simulink model "simulacion"  (R2019a)
settings: Solver=VariableStepAuto  StartTime=0.0  StopTime=25  RelTol=1e-3
values from neighbouring files (symbols this model uses):
  A = [1 -1.57039885123 1.27561332498 -0.484403368335 0.0761970646103]    [filtro.mat]
  B = [0.0185630106269 0.0742520425076 0.111378063761 0.0742520425076 0.0185630106269]    [filtro.mat]
  tm = 1.25531256352    [data_lineal.mat]    (also in modelo_1_orden_tiempo_muerto.m = 1.2620*dt25 - 0.2620*dt75; planta.mat)
libraries: cstblocks x17, simulink x9
settings Model: Creator=Juan P Velandia  LastModifiedBy=Juan P Velandia

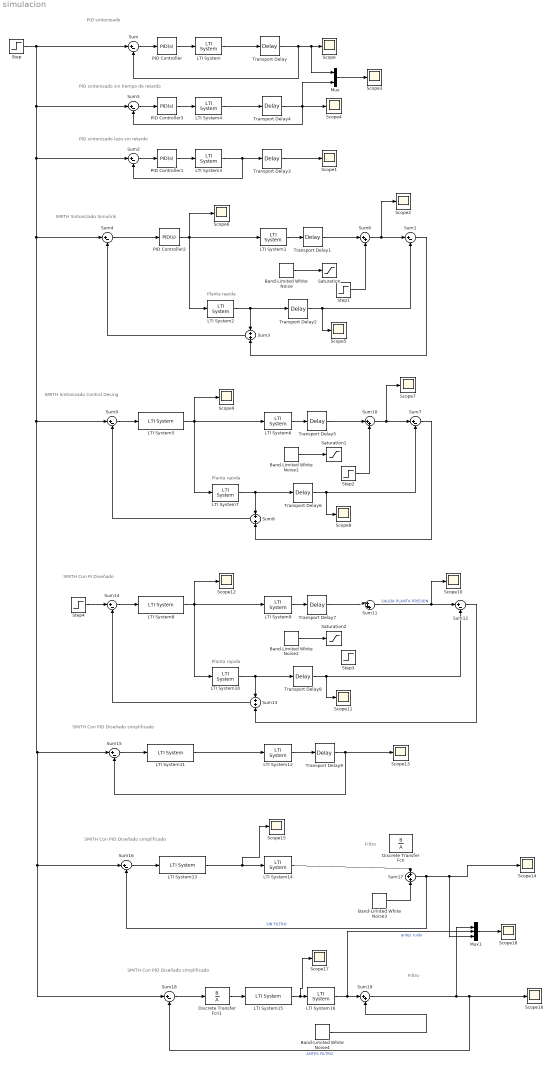
== system simulacion ==
  note: Filtro
  note: Planta rapida
  note: PID sintonizado
  note: PID sintonizado lazo sin retardo
  note: SMITH Sintonizado Simulink
  note: PID sintonizado sin tiempo de retardo
  note: Planta rapida
  note: SMITH Sintonizado Control Desing
  note: SMITH Con PI Diseñado
  note: Planta rapida
  note: SMITH Con PID Diseñado simplificado
  note: SMITH Con PID Diseñado simplificado
  note: Filtro
  note: SMITH Con PID Diseñado simplificado
  Band-Limited White Noise : simulink/Sources/Band-Limited White Noise  Cov=[0.1]  Ts=1  seed=[23341]
  Band-Limited White Noise1 : simulink/Sources/Band-Limited White Noise  Cov=[0.1]  Ts=1  seed=[23341]
  Band-Limited White Noise2 : simulink/Sources/Band-Limited White Noise  Cov=[0.1]  Ts=1  seed=[23341]
  Band-Limited White Noise3 : simulink/Sources/Band-Limited White Noise  Cov=[0.0008]  Ts=0.4  seed=[23341]
  Band-Limited White Noise4 : simulink/Sources/Band-Limited White Noise  Cov=[0.0008]  Ts=0.4  seed=[23341]
  Discrete Transfer Fcn : DiscreteTransferFcn  Numerator=B  Denominator=A
  Discrete Transfer Fcn1 : DiscreteTransferFcn  Numerator=B  Denominator=A
  LTI System{,1..2,6..7,9..10,12} (8 alike) : cstblocks/LTI System  sys=G  IC=[]
  LTI System11 : cstblocks/LTI System  sys=ceq  IC=[]
  LTI System13 : cstblocks/LTI System  sys=ceq_d  IC=[]
  LTI System14 : cstblocks/LTI System  sys=G_d  IC=[]
  LTI System15 : cstblocks/LTI System  sys=ceq_d  IC=[]
  LTI System16 : cstblocks/LTI System  sys=G_d  IC=[]
  LTI System3 : cstblocks/LTI System  sys=Gp1  IC=[]
  LTI System4 : cstblocks/LTI System  sys=Gp1  IC=[]
  LTI System5 : cstblocks/LTI System  sys=C  IC=[]
  LTI System8 : cstblocks/LTI System  sys=PI  IC=[]
  Mux : Mux  Inputs=2
  Mux1 : Mux  Inputs=3
  PID Controller : simulink/Continuous/PID Controller  Controller=PID  Form=Parallel  TimeDomain=Continuous-time  SampleTime=-1  IntegratorMethod=Forward Euler  FilterMethod=Forward Euler  ControllerParametersSource=internal  P=4249.87443519566  I=716.116002525779  D=-20348.5974264342  UseFilter=on  N=0.10676453447151  TunerSelectOption=Transfer Function Based (PID Tuner App)  InitialConditionSource=internal  InitialConditionForIntegrator=0  InitialConditionForFilter=0  DifferentiatorICPrevScaledInput=0  ExternalReset=none  TrackingMode=off  Kt=1  LimitOutput=off  UpperSaturationLimit=inf  LowerSaturationLimit=-inf  LinearizeAsGain=on  AntiWindupMode=none  Kb=1  POutMin=[]  POutMax=[]  IOutMin=[]  IOutMax=[]  DOutMin=[]  DOutMax=[]  NOutMin=[]  NOutMax=[]  SumOutMin=[]  SumOutMax=[]  SaturationOutMin=[]  SaturationOutMax=[]  PParamMin=[]  PParamMax=[]  IParamMin=[]  IParamMax=[]  DParamMin=[]  DParamMax=[]  NParamMin=[]  NParamMax=[]  KbParamMin=[]  KbParamMax=[]  KtParamMin=[]  KtParamMax=[]  KbOutMin=[]  KbOutMax=[]  KtOutMin=[]  KtOutMax=[]  IntegratorOutMin=[]  IntegratorOutMax=[]  FilterOutMin=[]  FilterOutMax=[]  SumI1OutMin=[]  SumI1OutMax=[]  SumI2OutMin=[]  SumI2OutMax=[]  SumI3OutMin=[]  SumI3OutMax=[]  SumI4OutMin=[]  SumI4OutMax=[]  SumDOutMin=[]  SumDOutMax=[]  DifferentiatorOutMin=[]  DifferentiatorOutMax=[]  FilterDiffOutCoefMin=[]  FilterDiffOutCoefMax=[]  ReciprocalOutMin=[]  ReciprocalOutMax=[]  SumDenOutMin=[]  SumDenOutMax=[]  SumNumOutMin=[]  SumNumOutMax=[]  DivideOutMin=[]  DivideOutMax=[]  IntegratorContinuousStateAttributes=''  IntegratorStateMustResolveToSignalObject=off  IntegratorRTWStateStorageClass=Auto  FilterContinuousStateAttributes=''  FilterStateMustResolveToSignalObject=off  FilterRTWStateStorageClass=Auto  ParallelPVariant=InternalParameters  IdealPVariant=Disabled  IVariant=InternalParameters  DVariant=InternalParameters  IntegratorVariant=Continuous  SatVariant=Disabled  AWVariant=Passthrough  PCopyVariant=Disabled  TRVariant=Disabled  FdbkBlocksVariant=Forward  IdealPFdbkVariant=Disabled  SatFdbkVariant=Disabled  DerivativeFilterVariant=ContFilter  NVariant=InternalParameters  NCopyVariant=Disabled  FilterICVariant=InternalICsFilter  IntegratorICVariant=InternalICs  ExternalResetVariant=Disabled  TRSumVariant=Passthrough  SumFdbkVariant=Disabled  SumVariant=Sum_PID
  PID Controller1 : simulink/Continuous/PID Controller  Controller=PID  Form=Parallel  TimeDomain=Continuous-time  SampleTime=-1  IntegratorMethod=Forward Euler  FilterMethod=Forward Euler  ControllerParametersSource=internal  P=5039.29122623723  I=1577.25793330017  D=-3349.52827806109  UseFilter=on  N=0.2130232522062  TunerSelectOption=Transfer Function Based (PID Tuner App)  InitialConditionSource=internal  InitialConditionForIntegrator=0  InitialConditionForFilter=0  DifferentiatorICPrevScaledInput=0  ExternalReset=none  TrackingMode=off  Kt=1  LimitOutput=off  UpperSaturationLimit=inf  LowerSaturationLimit=-inf  LinearizeAsGain=on  AntiWindupMode=none  Kb=1  POutMin=[]  POutMax=[]  IOutMin=[]  IOutMax=[]  DOutMin=[]  DOutMax=[]  NOutMin=[]  NOutMax=[]  SumOutMin=[]  SumOutMax=[]  SaturationOutMin=[]  SaturationOutMax=[]  PParamMin=[]  PParamMax=[]  IParamMin=[]  IParamMax=[]  DParamMin=[]  DParamMax=[]  NParamMin=[]  NParamMax=[]  KbParamMin=[]  KbParamMax=[]  KtParamMin=[]  KtParamMax=[]  KbOutMin=[]  KbOutMax=[]  KtOutMin=[]  KtOutMax=[]  IntegratorOutMin=[]  IntegratorOutMax=[]  FilterOutMin=[]  FilterOutMax=[]  SumI1OutMin=[]  SumI1OutMax=[]  SumI2OutMin=[]  SumI2OutMax=[]  SumI3OutMin=[]  SumI3OutMax=[]  SumI4OutMin=[]  SumI4OutMax=[]  SumDOutMin=[]  SumDOutMax=[]  DifferentiatorOutMin=[]  DifferentiatorOutMax=[]  FilterDiffOutCoefMin=[]  FilterDiffOutCoefMax=[]  ReciprocalOutMin=[]  ReciprocalOutMax=[]  SumDenOutMin=[]  SumDenOutMax=[]  SumNumOutMin=[]  SumNumOutMax=[]  DivideOutMin=[]  DivideOutMax=[]  IntegratorContinuousStateAttributes=''  IntegratorStateMustResolveToSignalObject=off  IntegratorRTWStateStorageClass=Auto  FilterContinuousStateAttributes=''  FilterStateMustResolveToSignalObject=off  FilterRTWStateStorageClass=Auto  ParallelPVariant=InternalParameters  IdealPVariant=Disabled  IVariant=InternalParameters  DVariant=InternalParameters  IntegratorVariant=Continuous  SatVariant=Disabled  AWVariant=Passthrough  PCopyVariant=Disabled  TRVariant=Disabled  FdbkBlocksVariant=Forward  IdealPFdbkVariant=Disabled  SatFdbkVariant=Disabled  DerivativeFilterVariant=ContFilter  NVariant=InternalParameters  NCopyVariant=Disabled  FilterICVariant=InternalICsFilter  IntegratorICVariant=InternalICs  ExternalResetVariant=Disabled  TRSumVariant=Passthrough  SumFdbkVariant=Disabled  SumVariant=Sum_PID
  PID Controller2 : simulink/Continuous/PID Controller  Controller=PID  Form=Parallel  TimeDomain=Continuous-time  SampleTime=-1  IntegratorMethod=Forward Euler  FilterMethod=Forward Euler  ControllerParametersSource=internal  P=5039.29122623723  I=1577.25793330017  D=-3349.52827806109  UseFilter=on  N=0.2130232522062  TunerSelectOption=Transfer Function Based (PID Tuner App)  InitialConditionSource=internal  InitialConditionForIntegrator=0  InitialConditionForFilter=0  DifferentiatorICPrevScaledInput=0  ExternalReset=none  TrackingMode=off  Kt=1  LimitOutput=off  UpperSaturationLimit=inf  LowerSaturationLimit=-inf  LinearizeAsGain=on  AntiWindupMode=none  Kb=1  POutMin=[]  POutMax=[]  IOutMin=[]  IOutMax=[]  DOutMin=[]  DOutMax=[]  NOutMin=[]  NOutMax=[]  SumOutMin=[]  SumOutMax=[]  SaturationOutMin=[]  SaturationOutMax=[]  PParamMin=[]  PParamMax=[]  IParamMin=[]  IParamMax=[]  DParamMin=[]  DParamMax=[]  NParamMin=[]  NParamMax=[]  KbParamMin=[]  KbParamMax=[]  KtParamMin=[]  KtParamMax=[]  KbOutMin=[]  KbOutMax=[]  KtOutMin=[]  KtOutMax=[]  IntegratorOutMin=[]  IntegratorOutMax=[]  FilterOutMin=[]  FilterOutMax=[]  SumI1OutMin=[]  SumI1OutMax=[]  SumI2OutMin=[]  SumI2OutMax=[]  SumI3OutMin=[]  SumI3OutMax=[]  SumI4OutMin=[]  SumI4OutMax=[]  SumDOutMin=[]  SumDOutMax=[]  DifferentiatorOutMin=[]  DifferentiatorOutMax=[]  FilterDiffOutCoefMin=[]  FilterDiffOutCoefMax=[]  ReciprocalOutMin=[]  ReciprocalOutMax=[]  SumDenOutMin=[]  SumDenOutMax=[]  SumNumOutMin=[]  SumNumOutMax=[]  DivideOutMin=[]  DivideOutMax=[]  IntegratorContinuousStateAttributes=''  IntegratorStateMustResolveToSignalObject=off  IntegratorRTWStateStorageClass=Auto  FilterContinuousStateAttributes=''  FilterStateMustResolveToSignalObject=off  FilterRTWStateStorageClass=Auto  ParallelPVariant=InternalParameters  IdealPVariant=Disabled  IVariant=InternalParameters  DVariant=InternalParameters  IntegratorVariant=Continuous  SatVariant=Disabled  AWVariant=Passthrough  PCopyVariant=Disabled  TRVariant=Disabled  FdbkBlocksVariant=Forward  IdealPFdbkVariant=Disabled  SatFdbkVariant=Disabled  DerivativeFilterVariant=ContFilter  NVariant=InternalParameters  NCopyVariant=Disabled  FilterICVariant=InternalICsFilter  IntegratorICVariant=InternalICs  ExternalResetVariant=Disabled  TRSumVariant=Passthrough  SumFdbkVariant=Disabled  SumVariant=Sum_PID
  PID Controller3 : simulink/Continuous/PID Controller  Controller=PID  Form=Parallel  TimeDomain=Continuous-time  SampleTime=-1  IntegratorMethod=Forward Euler  FilterMethod=Forward Euler  ControllerParametersSource=internal  P=5039.29122623723  I=1577.25793330017  D=-3349.52827806109  UseFilter=on  N=0.2130232522062  TunerSelectOption=Transfer Function Based (PID Tuner App)  InitialConditionSource=internal  InitialConditionForIntegrator=0  InitialConditionForFilter=0  DifferentiatorICPrevScaledInput=0  ExternalReset=none  TrackingMode=off  Kt=1  LimitOutput=off  UpperSaturationLimit=inf  LowerSaturationLimit=-inf  LinearizeAsGain=on  AntiWindupMode=none  Kb=1  POutMin=[]  POutMax=[]  IOutMin=[]  IOutMax=[]  DOutMin=[]  DOutMax=[]  NOutMin=[]  NOutMax=[]  SumOutMin=[]  SumOutMax=[]  SaturationOutMin=[]  SaturationOutMax=[]  PParamMin=[]  PParamMax=[]  IParamMin=[]  IParamMax=[]  DParamMin=[]  DParamMax=[]  NParamMin=[]  NParamMax=[]  KbParamMin=[]  KbParamMax=[]  KtParamMin=[]  KtParamMax=[]  KbOutMin=[]  KbOutMax=[]  KtOutMin=[]  KtOutMax=[]  IntegratorOutMin=[]  IntegratorOutMax=[]  FilterOutMin=[]  FilterOutMax=[]  SumI1OutMin=[]  SumI1OutMax=[]  SumI2OutMin=[]  SumI2OutMax=[]  SumI3OutMin=[]  SumI3OutMax=[]  SumI4OutMin=[]  SumI4OutMax=[]  SumDOutMin=[]  SumDOutMax=[]  DifferentiatorOutMin=[]  DifferentiatorOutMax=[]  FilterDiffOutCoefMin=[]  FilterDiffOutCoefMax=[]  ReciprocalOutMin=[]  ReciprocalOutMax=[]  SumDenOutMin=[]  SumDenOutMax=[]  SumNumOutMin=[]  SumNumOutMax=[]  DivideOutMin=[]  DivideOutMax=[]  IntegratorContinuousStateAttributes=''  IntegratorStateMustResolveToSignalObject=off  IntegratorRTWStateStorageClass=Auto  FilterContinuousStateAttributes=''  FilterStateMustResolveToSignalObject=off  FilterRTWStateStorageClass=Auto  ParallelPVariant=InternalParameters  IdealPVariant=Disabled  IVariant=InternalParameters  DVariant=InternalParameters  IntegratorVariant=Continuous  SatVariant=Disabled  AWVariant=Passthrough  PCopyVariant=Disabled  TRVariant=Disabled  FdbkBlocksVariant=Forward  IdealPFdbkVariant=Disabled  SatFdbkVariant=Disabled  DerivativeFilterVariant=ContFilter  NVariant=InternalParameters  NCopyVariant=Disabled  FilterICVariant=InternalICsFilter  IntegratorICVariant=InternalICs  ExternalResetVariant=Disabled  TRSumVariant=Passthrough  SumFdbkVariant=Disabled  SumVariant=Sum_PID
  Saturation : Saturate  UpperLimit=0.1  LowerLimit=-0.1
  Saturation1 : Saturate  UpperLimit=0.1  LowerLimit=-0.1
  Saturation2 : Saturate  UpperLimit=0.1  LowerLimit=-0.1
  Scope{,1..18} (19 alike) : Scope
  Step : Step  After=2.5  SampleTime=0
  Step1 : Step  Time=60  After=0.5  SampleTime=0
  Step2 : Step  Time=60  After=0.5  SampleTime=0
  Step3 : Step  Time=60  After=0.5  SampleTime=0
  Step4 : Step  After=2  SampleTime=0
  Sum{,1..2,4..5,7,9,12,14..16,18} (12 alike) : Sum  Inputs=|+-
  Sum10 : Sum  Inputs=|++
  Sum11 : Sum  Inputs=|+++
  Sum13 : Sum
  Sum17 : Sum  Inputs=+++
  Sum19 : Sum  Inputs=|++
  Sum3 : Sum
  Sum6 : Sum  Inputs=|++
  Sum8 : Sum
  Transport Delay{,1..9} (10 alike) : TransportDelay  DelayTime=tm
  wires:
  PID Controller/1 -> LTI System/1
  Sum/1 -> PID Controller/1
  LTI System/1 -> Transport Delay/1
  Transport Delay/1 -> Mux/1, Scope/1, Sum/2
  PID Controller2/1 -> Scope6/1, LTI System2/1, LTI System1/1
  LTI System1/1 -> Transport Delay1/1
  PID Controller1/1 -> LTI System3/1
  Sum2/1 -> PID Controller1/1
  LTI System3/1 -> Transport Delay3/1, Sum2/2
  Transport Delay1/1 -> Sum6/1
  Transport Delay2/1 -> Scope5/1, Sum1/2
  Transport Delay3/1 -> Scope1/1
  LTI System2/1 -> Transport Delay2/1, Sum3/1
  Sum1/1 -> Sum3/2
  Sum3/1 -> Sum4/2
  Sum4/1 -> PID Controller2/1
  Mux/1 -> Scope3/1
  Transport Delay4/1 -> Mux/2, Sum5/2, Scope4/1
  Sum5/1 -> PID Controller3/1
  PID Controller3/1 -> LTI System4/1
  LTI System4/1 -> Transport Delay4/1
  Band-Limited White Noise/1 -> Saturation/1
  Sum6/1 -> Scope2/1, Sum1/1
  Step1/1 -> Sum6/2
  Sum10/1 -> Scope7/1, Sum7/1
  Sum8/1 -> Sum9/2
  LTI System5/1 -> Scope9/1, LTI System7/1, LTI System6/1
  Transport Delay5/1 -> Sum10/1
  LTI System6/1 -> Transport Delay5/1
  Sum7/1 -> Sum8/2
  Band-Limited White Noise1/1 -> Saturation1/1
  LTI System7/1 -> Transport Delay6/1, Sum8/1
  Transport Delay6/1 -> Scope8/1, Sum7/2
  Sum9/1 -> LTI System5/1
  Step2/1 -> Sum10/2
  Sum11/1 -> Scope10/1, Sum12/1  "SALIDA PLANTA PRESION"
  Sum14/1 -> LTI System8/1
  Band-Limited White Noise2/1 -> Saturation2/1
  LTI System10/1 -> Transport Delay8/1, Sum13/1
  LTI System9/1 -> Transport Delay7/1
  Sum12/1 -> Sum13/2
  Transport Delay7/1 -> Sum11/1
  LTI System8/1 -> Scope12/1, LTI System10/1, LTI System9/1
  Transport Delay8/1 -> Scope11/1, Sum12/2
  Sum13/1 -> Sum14/2
  Step/1 -> Sum5/1, Sum18/1, Sum16/1, Sum15/1, Sum9/1, Sum4/1, Sum2/1, Sum/1
  Sum15/1 -> LTI System11/1
  LTI System11/1 -> LTI System12/1
  LTI System12/1 -> Transport Delay9/1
  Transport Delay9/1 -> Scope13/1, Sum15/2
  Sum16/1 -> LTI System13/1
  LTI System13/1 -> Scope15/1, LTI System14/1
  Sum17/1 -> Mux1/3, Scope14/1, Sum16/2  "SIN FILTRO"
  LTI System14/1 -> Sum17/1
  LTI System15/1 -> Scope17/1, LTI System16/1
  Sum19/1 -> Mux1/1, Sum18/2, Scope16/1  "ANTES FILTRO"
  LTI System16/1 -> Mux1/2, Sum19/1  "antes ruido"
  Mux1/1 -> Scope18/1
  Band-Limited White Noise4/1 -> Sum19/2
  Band-Limited White Noise3/1 -> Sum17/3
  Sum18/1 -> Discrete Transfer Fcn1/1
  Discrete Transfer Fcn1/1 -> LTI System15/1
  Step4/1 -> Sum14/1
